simulink library "moving_average_filter"  (R2025b)
settings: Solver=VariableStepAuto  StartTime=0.0  StopTime=10.0  RelTol=1e-3
undefined symbols (not defined in the file): ts_afe
libraries: simulink x1
settings Model: Creator=dbagn  LastModifiedBy=dbagn
settings SFSimCC: SimCustomHeaderCode=|
  | #include "dsmavgflt.h"
  | #include "dsmavgflt_simulink.h"
  | #include "mavgflt.h"
  | #include "mavgflt_simulink.h"
  | #include "mavgflts.h"
  | #include "mavgflts_simulink.h"
settings SFSimCC: SimUserSources=|
  | "dsmavgflt_simulink.c"
  | "dsmavgflt.c"
  | "mavgflts_simulink.c"
  | "mavgflts.c"
  | "mavgflt_simulink.c"
  | "mavgflt.c"
settings SFSimCC: SimUserIncludeDirs=|
  | include
  | src

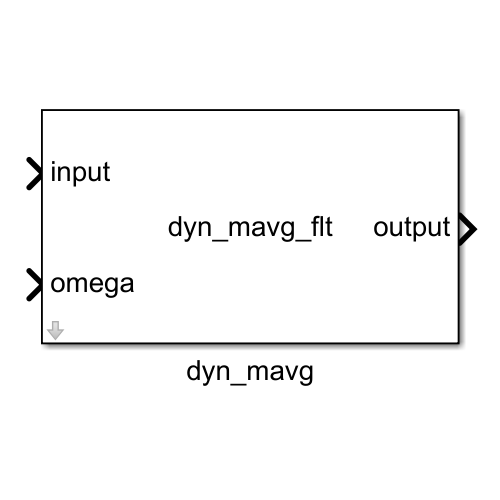
[thumbnail: Simulink's stored preview of the top-level diagram]
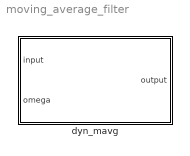
== system moving_average_filter ==
  dyn_mavg : Subsystem  mask{ts=ts_afe, start_delay=0.0125}
      mask prompts: ts "sampling time (s)"; start_delay "start_delay (s)"
      mask Display:
      | disp('dyn_mavg_flt');
      | port_label('input', 1, 'input');
      | port_label('input', 2, 'omega');
      | port_label('output', 1, 'output');

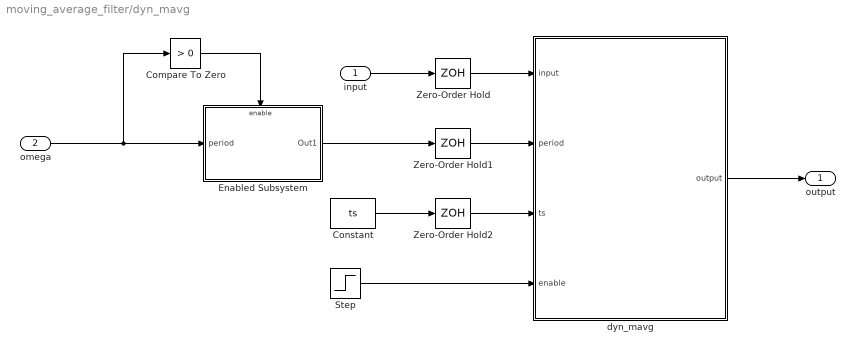
== system moving_average_filter/dyn_mavg ==
  input : Inport
  omega : Inport  Port=2
  Compare To Zero : simulink/Logic and Bit Operations/Compare To Zero  relop=>  OutDataTypeStr=boolean
  Constant : Constant  Value=ts
  Enabled Subsystem : Subsystem  TreatAsAtomicUnit=on
  Step : Step  Time=start_delay
  Zero-Order Hold : ZeroOrderHold  SampleTime=-1
  Zero-Order Hold1 : ZeroOrderHold  SampleTime=-1
  Zero-Order Hold2 : ZeroOrderHold  SampleTime=-1
  dyn_mavg : MATLAB Function  TreatAsAtomicUnit=on
  output : Outport
  wires:
  dyn_mavg/1(output) -> output/1
  Compare To Zero/1 -> Enabled Subsystem/Enable
  omega/1 -> Compare To Zero/1, Enabled Subsystem/1(period)
  input/1 -> Zero-Order Hold/1
  Zero-Order Hold/1 -> dyn_mavg/1(input)
  Enabled Subsystem/1(Out1) -> Zero-Order Hold1/1
  Constant/1 -> Zero-Order Hold2/1
  Zero-Order Hold2/1 -> dyn_mavg/3(ts)
  Zero-Order Hold1/1 -> dyn_mavg/2(period)
  Step/1 -> dyn_mavg/4(enable)

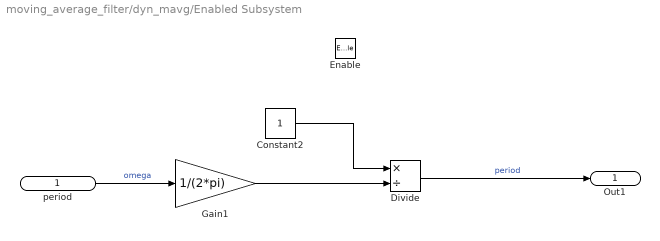
== system moving_average_filter/dyn_mavg/Enabled Subsystem ==
  period : Inport
  Enable : EnablePort
  Constant2 : Constant
  Divide : Product  Inputs=*/
  Gain1 : Gain  Gain=1/(2*pi)
  Out1 : Outport
  wires:
  Constant2/1 -> Divide/1
  period/1 -> Gain1/1  "omega"
  Gain1/1 -> Divide/2
  Divide/1 -> Out1/1  "period"

== matlab function moving_average_filter/dyn_mavg/dyn_mavg ==
  data: input input; output output; period input; ts input; enable input
function output = dyn_mavg(input, period, ts, enable)
% dyn_mavg  
% s = shorter
% l = longer

    persistent buffer_s buffer_l idx_s idx_l Nmax sum_buffer_s sum_buffer_l

    if isempty(buffer_s)
        Nmax = 1600;           
        buffer_s = zeros(1, Nmax);
        buffer_l = zeros(1, Nmax);
        idx_s = 1;
        idx_l = 1;
        sum_buffer_s = 0;
        sum_buffer_l = 0;
    end
    if enable
        length_period_f = period / ts;
        length_period_s = floor(length_period_f);
        length_period_l = length_period_s + 1;
        frac = length_period_f - length_period_s; % fractional part
    
        % Indice campione più vecchio
        old_idx_s = mod(idx_s - length_period_s - 1, Nmax) + 1;
        old_idx_l = mod(idx_l - length_period_l - 1, Nmax) + 1;
        xn_s = buffer_s(old_idx_s);
        xn_l = buffer_l(old_idx_l);
    
        % Aggiorna somma
        sum_buffer_s = sum_buffer_s - xn_s + input;
        sum_buffer_l = sum_buffer_l - xn_l + input;
        buffer_s(idx_s) = input;
        buffer_l(idx_l) = input;
    
        % Calcola output pesato
        output = (1 - frac) * sum_buffer_s/length_period_s + frac * sum_buffer_l/length_period_l;
    
        % Aggiorna indice circolare
        idx_s = mod(idx_s, Nmax) + 1;
        idx_l = mod(idx_l, Nmax) + 1;
    else
        output = 0;
    end
end
